simulink model "SVPWM_simulation"  (R2023a)
settings: Solver=FixedStepAuto  StartTime=0.0  StopTime=0.1  RelTol=1e-3
values from neighbouring files (symbols this model uses):
  K_xyz = sqrt(3)*T_sw/V_dc    [SVPWM.m]
  T_sw = 1/f_sw    (= 0.0001)    [SVPWM.m]
  V_dc = 500    [SVPWM.m]
libraries: simulink x4, spsSeriesRLCBranchLib x3, spsVoltageMeasurementLib x3, spsDCVoltageSourceLib x2, spsGroundLib x1, spsUniversalBridgeLib x1, spsabctoAlphaBetaZeroLib x1, sps_lib x1
settings Model: Creator=11048  LastModifiedBy=11048

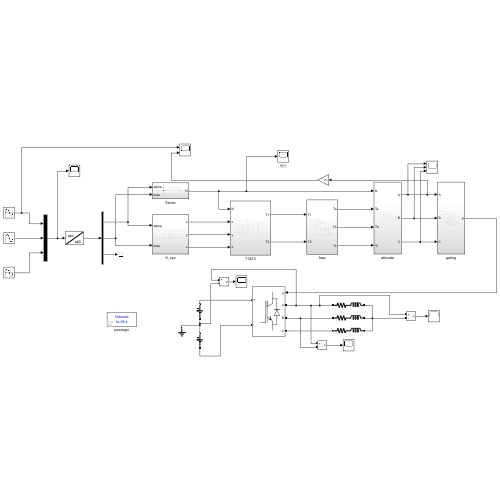
[thumbnail: Simulink's stored preview of the top-level diagram]
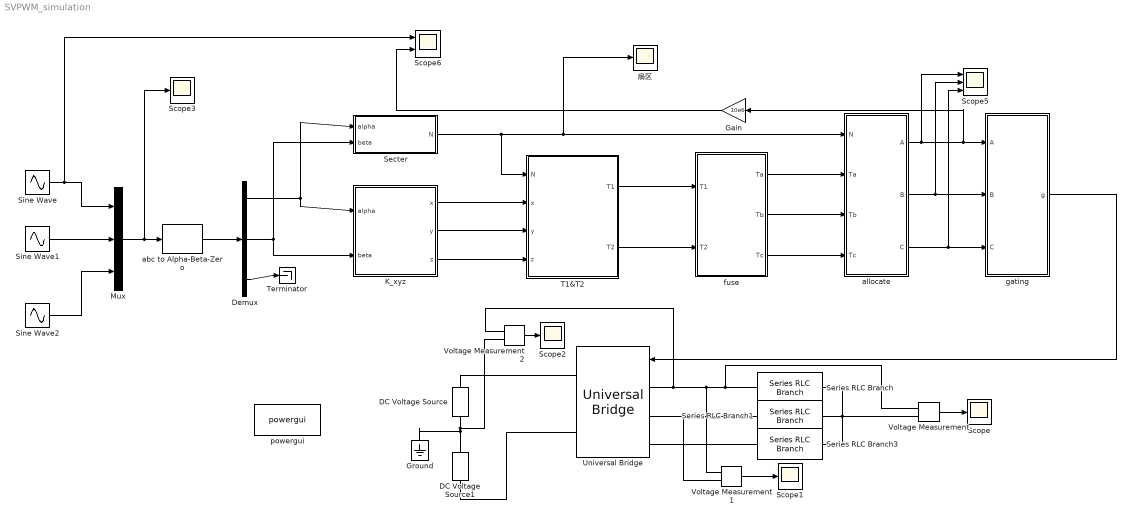
== system SVPWM_simulation ==
  DC Voltage Source : spsDCVoltageSourceLib/DC Voltage Source  Amplitude=V_dc/2  Measurements=None
  DC Voltage Source1 : spsDCVoltageSourceLib/DC Voltage Source  Amplitude=V_dc/2  Measurements=None
  Demux : Demux  Outputs=3
  Gain : Gain  Gain=10e6
  Ground : spsGroundLib/Ground  LConnTagsString=a
  K_xyz : Subsystem
  Mux : Mux  Inputs=3
  Scope{,1..3} (4 alike) : Scope
  Scope5 : Scope  NumInputPorts=3
  Scope6 : Scope  NumInputPorts=2
  Secter : Subsystem
  Series RLC Branch : spsSeriesRLCBranchLib/Series RLC Branch  LConnTagsString=__new0  RConnTagsString=__new0  BranchType=RL  Resistance=1  Inductance=1e-3  SetiL0=off  InitialCurrent=0  Capacitance=1e-6  Setx0=off  InitialVoltage=0  Measurements=None
  Series RLC Branch1 : spsSeriesRLCBranchLib/Series RLC Branch  LConnTagsString=__new0  RConnTagsString=__new0  BranchType=RL  Resistance=1  Inductance=1e-3  SetiL0=off  InitialCurrent=0  Capacitance=1e-6  Setx0=off  InitialVoltage=0  Measurements=None
  Series RLC Branch3 : spsSeriesRLCBranchLib/Series RLC Branch  LConnTagsString=__new0  RConnTagsString=__new0  BranchType=RL  Resistance=1  Inductance=1e-3  SetiL0=off  InitialCurrent=0  Capacitance=1e-6  Setx0=off  InitialVoltage=0  Measurements=None
  Sine Wave : Sin  Amplitude=220*sqrt(2)/sqrt(3)  Frequency=50*2*pi  SampleTime=0
  Sine Wave1 : Sin  Amplitude=220*sqrt(2)/sqrt(3)  Frequency=50*2*pi  Phase=-(2/3)*pi  SampleTime=0
  Sine Wave2 : Sin  Amplitude=220*sqrt(2)/sqrt(3)  Frequency=50*2*pi  Phase=(2/3)*pi  SampleTime=0
  T1&T2 : Subsystem
  Terminator : Terminator
  Universal Bridge : spsUniversalBridgeLib/Universal Bridge  Arms=3  SnubberResistance=1e5  SnubberCapacitance=inf  Device=IGBT / Diodes  Ron=1e-3  Lon=0  ForwardVoltages="[  0  0  ]"  ForwardVoltage=0  GTOparameters=[ 10e-6 , 20e-6 ]  IGBTparameters=[ 1e-6 , 2e-6 ]  Measurements=None  Measurements_2=None  converterType=Rectifier
  Voltage Measurement : spsVoltageMeasurementLib/Voltage Measurement  PhasorSimulation=off  OutputType=Complex  PSBequivalent=0
  Voltage Measurement1 : spsVoltageMeasurementLib/Voltage Measurement  PhasorSimulation=off  OutputType=Complex  PSBequivalent=0
  Voltage Measurement2 : spsVoltageMeasurementLib/Voltage Measurement  PhasorSimulation=off  OutputType=Complex  PSBequivalent=0
  abc to Alpha-Beta-Zero : spsabctoAlphaBetaZeroLib/abc to Alpha-Beta-Zero
  allocate : Subsystem
  fuse : Subsystem
  gating : Subsystem
  powergui : sps_lib/powergui  Priority=1  SimulationMode=Discrete  SampleTime=T_sw/10  frequency=60  Iterations=50  frequencyindice=0  Pbase=100e6  ErrMax=1e-4  UnitsV=kV  UnitsW=MW  buscounter=0  FunctionMessages=off  echomessages=off  EnableUseOfTLC=off  CurrentSourceSwitches=off  DisableSnubberDevices=off  DisableRonSwitches=off  DisableVfSwitches=off  DisplayEquations=off  AutomaticDiscreteSolvers=off  SolverType=Tustin/Backward Euler (TBE)  Interpol=off  ExternalGateDelay=off  methode=off  Ts=100  x0status=blocks  SPID=on  SwTol=0  HookPort=off  NonlinearTolerance=1e-4  nMaxIteration=100  ContinueOnMaxIteration=off  RestoreLinks=warning  ResistiveCurrentMeasurement=off  Frange=[0:2:500]  Ylog=off  Xlog=on  ShowGrid=off  save=off  variable=ZData  structure=0  ZoomFFT=off  StartTime=0.0  cycles=1  DisplayStyle=1  fundamental=60  FreqAxis=off  MaxFrequency=1000  frequencyindicesteady=1  RmsSteady=1  display=off
  扇区 : Scope
  wires:
  Secter/1(N) -> 扇区/1, allocate/1(N), T1&T2/1(N)
  K_xyz/2(y) -> T1&T2/3(y)
  K_xyz/1(x) -> T1&T2/2(x)
  K_xyz/3(z) -> T1&T2/4(z)
  T1&T2/1(" T1") -> fuse/1(T1)
  T1&T2/2(T2) -> fuse/2(T2)
  fuse/2(Tb) -> allocate/3(Tb)
  fuse/1(Ta) -> allocate/2(Ta)
  fuse/3(Tc) -> allocate/4(Tc)
  allocate/1(A) -> Scope5/1, Gain/1, gating/1(A)
  allocate/2(B) -> gating/2(B), Scope5/2
  allocate/3(C) -> Scope5/3, gating/3(C)
  Mux/1 -> Scope3/1, abc to Alpha-Beta-Zero/1
  Demux/3 -> Terminator/1
  abc to Alpha-Beta-Zero/1 -> Demux/1
  Sine Wave/1 -> Scope6/1, Mux/1
  Sine Wave1/1 -> Mux/2
  Sine Wave2/1 -> Mux/3
  gating/1(g) -> Universal Bridge/1
  Voltage Measurement/1 -> Scope/1
  Voltage Measurement1/1 -> Scope1/1
  Voltage Measurement2/1 -> Scope2/1
  Demux/1 -> K_xyz/1(alpha), Secter/1(alpha)
  Demux/2 -> K_xyz/2(beta), Secter/2(beta)
  Gain/1 -> Scope6/2
  connections:
  DC Voltage Source/LConn1 -- Ground/LConn1 -- DC Voltage Source1/RConn1 -- Voltage Measurement2/LConn2
  DC Voltage Source/RConn1 -- Universal Bridge/RConn1
  DC Voltage Source1/LConn1 -- Universal Bridge/RConn2
  Series RLC Branch/RConn1 -- Voltage Measurement/LConn2 -- Series RLC Branch1/RConn1 -- Series RLC Branch3/RConn1
  Series RLC Branch/LConn1 -- Voltage Measurement/LConn1 -- Voltage Measurement1/LConn1 -- Voltage Measurement2/LConn1 -- Universal Bridge/LConn1
  Universal Bridge/LConn2 -- Voltage Measurement1/LConn2 -- Series RLC Branch1/LConn1
  Universal Bridge/LConn3 -- Series RLC Branch3/LConn1

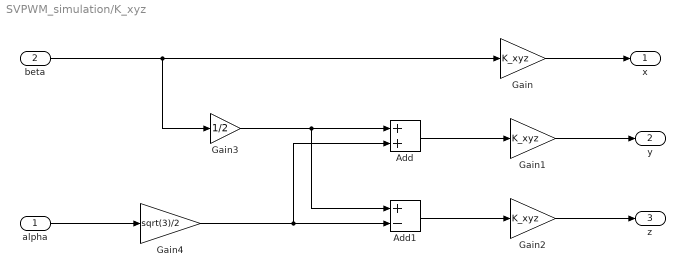
== system SVPWM_simulation/K_xyz ==
  alpha : Inport
  beta : Inport  Port=2
  Add : Sum
  Add1 : Sum  Inputs=+-
  Gain : Gain  Gain=K_xyz
  Gain1 : Gain  Gain=K_xyz
  Gain2 : Gain  Gain=K_xyz
  Gain3 : Gain  Gain=1/2
  Gain4 : Gain  Gain=sqrt(3)/2
  x : Outport
  y : Outport  Port=2
  z : Outport  Port=3
  wires:
  Gain/1 -> x/1
  Gain1/1 -> y/1
  Gain2/1 -> z/1
  alpha/1 -> Gain4/1
  Gain4/1 -> Add/2, Add1/2
  beta/1 -> Gain3/1, Gain/1
  Gain3/1 -> Add1/1, Add/1
  Add/1 -> Gain1/1
  Add1/1 -> Gain2/1

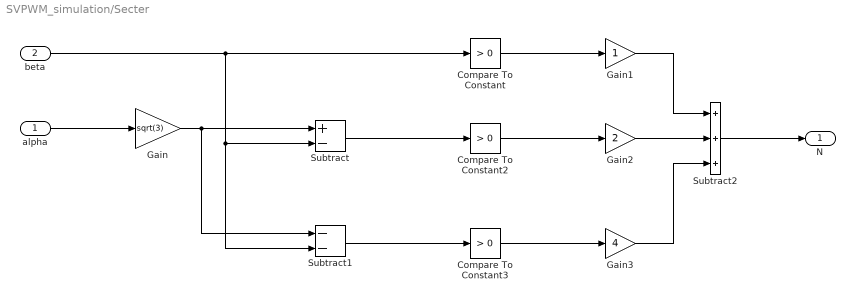
== system SVPWM_simulation/Secter ==
  alpha : Inport
  beta : Inport  Port=2
  Compare To Constant : simulink/Logic and Bit Operations/Compare To Constant  relop=>  const=0  OutDataTypeStr=boolean
  Compare To Constant2 : simulink/Logic and Bit Operations/Compare To Constant  relop=>  const=0  OutDataTypeStr=boolean
  Compare To Constant3 : simulink/Logic and Bit Operations/Compare To Constant  relop=>  const=0  OutDataTypeStr=boolean
  Gain : Gain  Gain=sqrt(3)
  Gain1 : Gain
  Gain2 : Gain  Gain=2
  Gain3 : Gain  Gain=4
  Subtract : Sum  Inputs=+-
  Subtract1 : Sum  Inputs=--
  Subtract2 : Sum  Inputs=+++
  N : Outport
  wires:
  Gain/1 -> Subtract1/1, Subtract/1
  Subtract/1 -> Compare To Constant2/1
  beta/1 -> Subtract1/2, Subtract/2, Compare To Constant/1
  alpha/1 -> Gain/1
  Subtract1/1 -> Compare To Constant3/1
  Compare To Constant/1 -> Gain1/1
  Compare To Constant2/1 -> Gain2/1
  Compare To Constant3/1 -> Gain3/1
  Gain1/1 -> Subtract2/1
  Gain2/1 -> Subtract2/2
  Gain3/1 -> Subtract2/3
  Subtract2/1 -> N/1

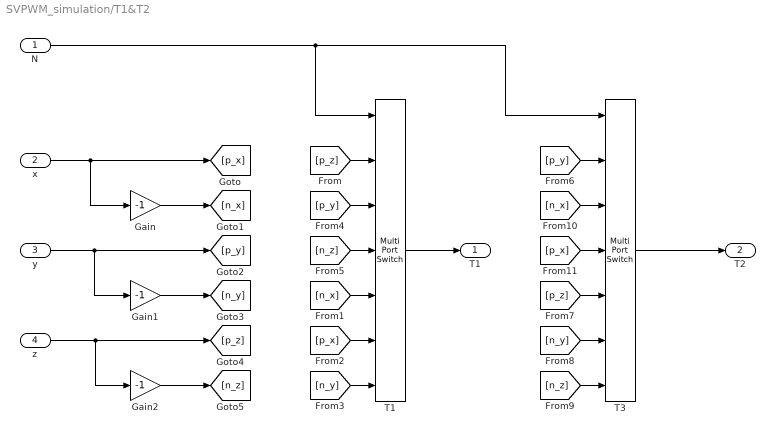
== system SVPWM_simulation/T1&T2 ==
  N : Inport
  x : Inport  Port=2
  y : Inport  Port=3
  z : Inport  Port=4
  Gain : Gain  Gain=-1
  Gain1 : Gain  Gain=-1
  Gain2 : Gain  Gain=-1
  T1 : MultiPortSwitch  Inputs=6  SaturateOnIntegerOverflow=off  InputSameDT=off
  T3 : MultiPortSwitch  Inputs=6  SaturateOnIntegerOverflow=off  InputSameDT=off
  " T1" : Outport
  T2 : Outport  Port=2
  wires:
  x/1 -> Gain/1, [p_x]
  T1/1 -> " T1"/1
  T3/1 -> T2/1
  y/1 -> Gain1/1, [p_y]
  z/1 -> Gain2/1, [p_z]
  Gain1/1 -> [n_y]
  Gain2/1 -> [n_z]
  [p_z] -> T1/2
  [p_y] -> T1/3
  [n_z] -> T1/4
  Gain/1 -> [n_x]
  [n_x] -> T1/5
  [p_x] -> T1/6
  [n_y] -> T1/7
  [n_z] -> T3/7
  [n_y] -> T3/6
  [p_z] -> T3/5
  [p_x] -> T3/4
  [n_x] -> T3/3
  [p_y] -> T3/2
  N/1 -> T3/1, T1/1

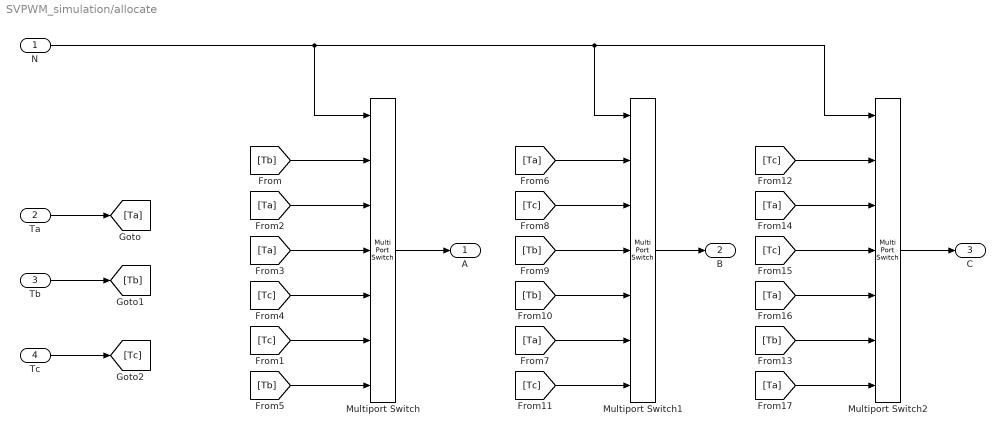
== system SVPWM_simulation/allocate ==
  N : Inport
  Ta : Inport  Port=2
  Tb : Inport  Port=3
  Tc : Inport  Port=4
  Multiport Switch : MultiPortSwitch  Inputs=6  SaturateOnIntegerOverflow=off  InputSameDT=off
  Multiport Switch1 : MultiPortSwitch  Inputs=6  SaturateOnIntegerOverflow=off  InputSameDT=off
  Multiport Switch2 : MultiPortSwitch  Inputs=6  SaturateOnIntegerOverflow=off  InputSameDT=off
  A : Outport
  B : Outport  Port=2
  C : Outport  Port=3
  wires:
  Ta/1 -> [Ta]
  Tb/1 -> [Tb]
  Tc/1 -> [Tc]
  [Tb] -> Multiport Switch/2
  [Ta] -> Multiport Switch/3
  [Ta] -> Multiport Switch/4
  [Tc] -> Multiport Switch/5
  [Tc] -> Multiport Switch/6
  [Tb] -> Multiport Switch/7
  Multiport Switch/1 -> A/1
  [Ta] -> Multiport Switch1/6
  [Tc] -> Multiport Switch1/7
  [Tb] -> Multiport Switch1/5
  [Tc] -> Multiport Switch1/3
  [Tb] -> Multiport Switch1/4
  [Ta] -> Multiport Switch1/2
  Multiport Switch2/1 -> C/1
  [Tb] -> Multiport Switch2/6
  [Ta] -> Multiport Switch2/7
  [Ta] -> Multiport Switch2/5
  [Ta] -> Multiport Switch2/3
  [Tc] -> Multiport Switch2/4
  [Tc] -> Multiport Switch2/2
  Multiport Switch1/1 -> B/1
  N/1 -> Multiport Switch/1, Multiport Switch2/1, Multiport Switch1/1

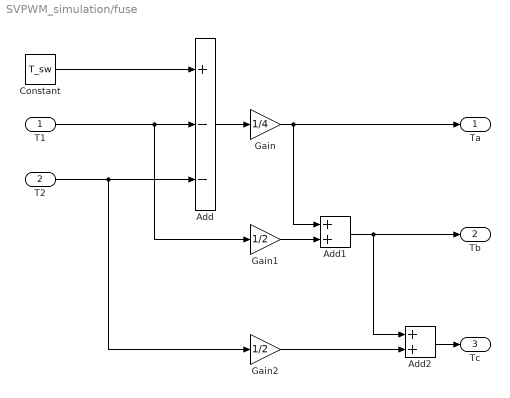
== system SVPWM_simulation/fuse ==
  T1 : Inport
  T2 : Inport  Port=2
  Add : Sum  Inputs=+--
  Add1 : Sum
  Add2 : Sum
  Constant : Constant  Value=T_sw
  Gain : Gain  Gain=1/4
  Gain1 : Gain  Gain=1/2
  Gain2 : Gain  Gain=1/2
  Ta : Outport
  Tb : Outport  Port=2
  Tc : Outport  Port=3
  wires:
  T2/1 -> Gain2/1, Add/3
  Constant/1 -> Add/1
  Add/1 -> Gain/1
  Gain/1 -> Ta/1, Add1/1
  Gain1/1 -> Add1/2
  Add1/1 -> Add2/1, Tb/1
  Add2/1 -> Tc/1
  Gain2/1 -> Add2/2
  T1/1 -> Add/2, Gain1/1

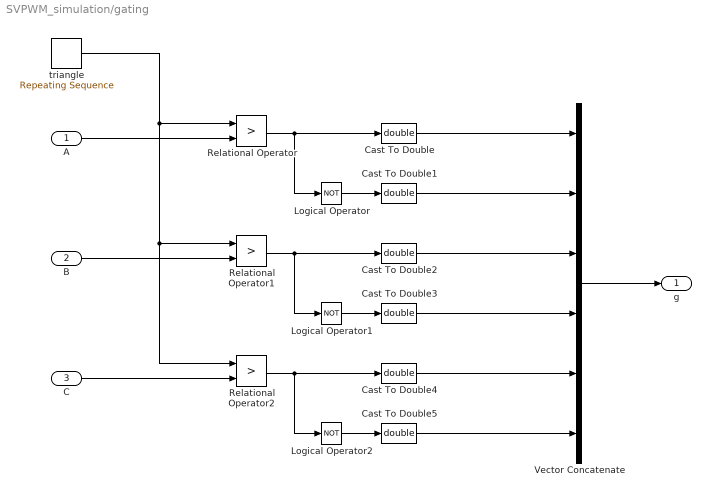
== system SVPWM_simulation/gating ==
  A : Inport
  B : Inport  Port=2
  C : Inport  Port=3
  Cast To Double{,1..5} (6 alike) : DataTypeConversion  OutDataTypeStr=double  SaturateOnIntegerOverflow=off  RndMeth=Floor
  Logical Operator : Logic  Operator=NOT  AllPortsSameDT=off  OutDataTypeStr=boolean
  Logical Operator1 : Logic  Operator=NOT  AllPortsSameDT=off  OutDataTypeStr=boolean
  Logical Operator2 : Logic  Operator=NOT  AllPortsSameDT=off  OutDataTypeStr=boolean
  Relational Operator : RelationalOperator  Operator=>  OutDataTypeStr=boolean  RndMeth=Simplest  InputSameDT=off
  Relational Operator1 : RelationalOperator  Operator=>  OutDataTypeStr=boolean  RndMeth=Simplest  InputSameDT=off
  Relational Operator2 : RelationalOperator  Operator=>  OutDataTypeStr=boolean  RndMeth=Simplest  InputSameDT=off
  Vector Concatenate : Concatenate  NumInputs=6
  triangle : simulink/Sources/Repeating Sequence  rep_seq_t=[0 T_sw/2 T_sw]  rep_seq_y=[0 T_sw/2 0]
  g : Outport
  wires:
  C/1 -> Relational Operator2/2
  B/1 -> Relational Operator1/2
  A/1 -> Relational Operator/2
  triangle/1 -> Relational Operator/1, Relational Operator2/1, Relational Operator1/1
  Cast To Double1/1 -> Vector Concatenate/2
  Relational Operator/1 -> Logical Operator/1, Cast To Double/1
  Logical Operator/1 -> Cast To Double1/1
  Logical Operator1/1 -> Cast To Double3/1
  Relational Operator1/1 -> Logical Operator1/1, Cast To Double2/1
  Cast To Double3/1 -> Vector Concatenate/4
  Logical Operator2/1 -> Cast To Double5/1
  Relational Operator2/1 -> Logical Operator2/1, Cast To Double4/1
  Cast To Double5/1 -> Vector Concatenate/6
  Cast To Double/1 -> Vector Concatenate/1
  Cast To Double2/1 -> Vector Concatenate/3
  Cast To Double4/1 -> Vector Concatenate/5
  Vector Concatenate/1 -> g/1
